simulink model "simulink_example_stateflow"  (R2014b)
settings: Solver=FixedStepDiscrete  StartTime=0.0  StopTime=inf  FixedStep=0.1  RelTol=1e-3
undefined symbols (not defined in the file or in its folder): simulink_example_config_stateflow
libraries: PaPI x2
settings Model: Creator=sven  LastModifiedBy=sven
settings OptimizationCC: OptimizeModelRefInitCode=on  LifeSpan=Inf
settings DebuggingCC: UnderspecifiedInitializationDetection=Classic  MergeDetectMultiDrivingBlocksExec=none  StateNameClashWarn=warning
settings RTWCC: SystemTargetFile=ert_linux.tlc  MakeCommand="make_rtw OPTS=\"-DWITH_HW=1\""  TemplateMakefile=ert_linux.tmf  Description=Linux Embedded Coder  ProcessScript=ert_linux_make_rtw_hook  TargetLang=C++
settings RTWCC: CustomInclude=|
  | /usr/local/MATLAB/R2014b/sys/os/glnxa64/
  | /usr/lib/x86_64-linux-gnu/
  | /usr/include/
settings RTWCC: CustomLibrary=|
  | libstdc++.so.6
  | libgcc_s.so.1
  | libgfortran.so.3
  | libdl.so
  | libboost_system.so
  | libboost_thread.so
  | libboost_signals.so
settings CodeAppCC: IgnoreCustomStorageClasses=off
settings STFCustomTargetCC: ModelReferenceCompliant=off  CombineOutputUpdateFcns=on  ERTCustomFileBanners=on  SupportContinuousTime=off  SupportNonInlinedSFcns=off  MATLABClassNameForMDSCustomization=Simulink.SoftwareTarget.ERTCustomization  GRTInterface=off  SystemTargetFile=ert_linux.tlc
settings ERTTargetCC: ModelReferenceCompliant=off  ParMdlRefBuildCompliant=off  CompOptLevelCompliant=off  ConcurrentExecutionCompliant=off  ERTFirstTimeCompliant=off  ModelStepFunctionPrototypeControlCompliant=off  CPPClassGenCompliant=off  ExtMode=on  InlinedParameterPlacement=NonHierarchical  ERTCustomFileTemplate=ert_linux_file_process.tlc

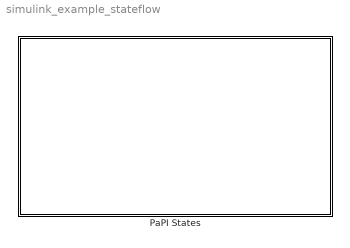
== system simulink_example_stateflow ==
  PaPI States : Stateflow chart  TreatAsAtomicUnit=on

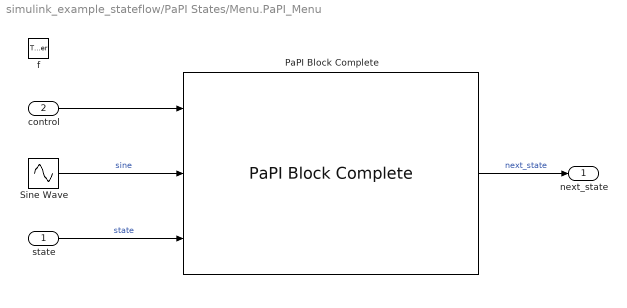
== system simulink_example_stateflow/PaPI States/Menu.PaPI_Menu ==
  state : Inport
  control : Inport  Port=2
  f : TriggerPort  TriggerType=function-call  StatesWhenEnabling=reset  SampleTime=0.1
      settings: CopyFcn=Stateflow.SLINSF.SimulinkMan.removeBlockPreDeleteFcn  PreDeleteFcn=Stateflow.SLINSF.SimulinkMan.unsafePredeleteFcn
  PaPI Block Complete : PaPI/PaPI Block Complete  amount_parameters=[1]  define_inputs=[1,1]  split_inputs=[1,1]  json_string=simulink_example_config_stateflow(1,1)  UDPLocalPort=20001  UDPRemotePort=20000  UDPRemoteIP='127.0.0.1'  output_size=200  sample_time=-1
  Sine Wave : Sin
  next_state : Outport
  wires:
  PaPI Block Complete/1 -> next_state/1  "next_state"
  Sine Wave/1 -> PaPI Block Complete/2  "sine"
  state/1 -> PaPI Block Complete/3  "state"
  control/1 -> PaPI Block Complete/1

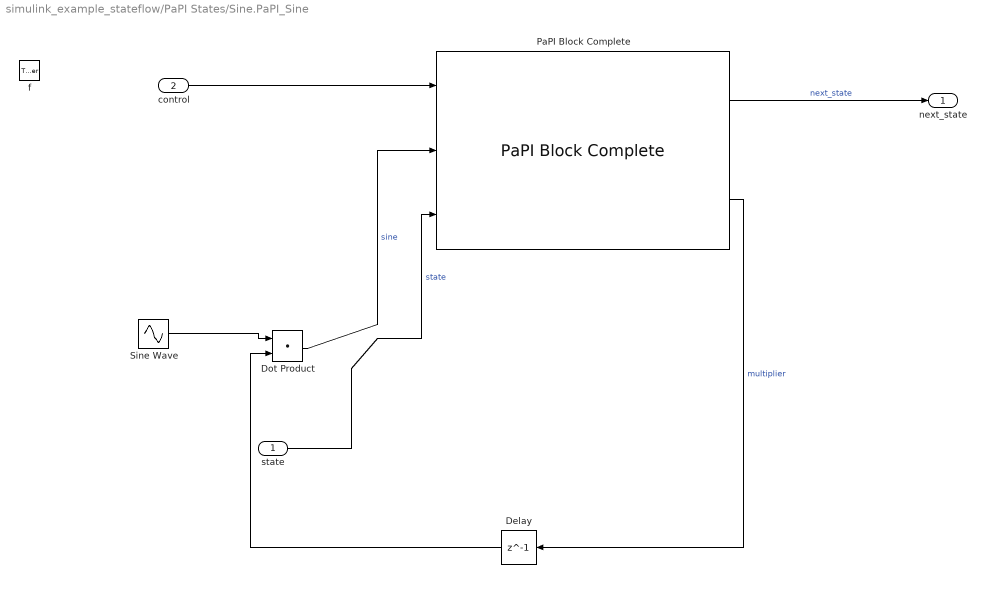
== system simulink_example_stateflow/PaPI States/Sine.PaPI_Sine ==
  state : Inport
  control : Inport  Port=2
  f : TriggerPort  TriggerType=function-call  StatesWhenEnabling=reset
      settings: CopyFcn=Stateflow.SLINSF.SimulinkMan.removeBlockPreDeleteFcn  PreDeleteFcn=Stateflow.SLINSF.SimulinkMan.unsafePredeleteFcn
  Delay : Delay  DelayLength=1
  Dot Product : DotProduct  InputSameDT=on  OutDataTypeStr=Inherit: Inherit via internal rule
  PaPI Block Complete : PaPI/PaPI Block Complete  amount_parameters=[1,1]  define_inputs=[1,1]  split_inputs=[1,1]  json_string=simulink_example_config_stateflow(2,1)  UDPLocalPort=20001  UDPRemotePort=20000  UDPRemoteIP='127.0.0.1'  output_size=200  sample_time=-1
  Sine Wave : Sin
  next_state : Outport
  wires:
  Sine Wave/1 -> Dot Product/1
  Dot Product/1 -> PaPI Block Complete/2  "sine"
  PaPI Block Complete/2 -> Delay/1  "multiplier"
  Delay/1 -> Dot Product/2
  PaPI Block Complete/1 -> next_state/1  "next_state"
  state/1 -> PaPI Block Complete/3  "state"
  control/1 -> PaPI Block Complete/1

== stateflow chart simulink_example_stateflow/PaPI States ==
  state Menu
    entry: state=1, [next_state] = PaPI_Menu(state,1),
    during: [next_state] = PaPI_Menu(state,0)
    exit: [next_state] = PaPI_Menu(state,2)
    state next_state  = PaPI_Menu(state,control) [function]
  state Sine
    entry: state=2, [next_state] = PaPI_Sine(state, 1)
    during: [next_state] = PaPI_Sine(state, 0)
    exit: [next_state] = PaPI_Sine(state, 2)
    state next_state  = PaPI_Sine(state,control) [function]
  (default) -> Menu
  Menu -> Sine : [next_state==2]
  Sine -> Menu : [next_state==1]
  data: next_state function_output; state function_input; control function_input; state function_input; control function_input; next_state function_output; state local double; next_state local double
